simulink model "reichardt_array_EMD"  (R2018b)
settings: Solver=ode45  StartTime=0.0  StopTime=setStopTime  FixedStep=0.0005  RelTol=1e-3  EnableMultiTasking=on
model workspace (MAT data in the model file):
  bodyAmp = 0
  bodyPhase = 0
  freq = 628.318530718
  headAmp = 0
  headPhase = 0
  imageData = [0.00303351691359 0.00909998476947 0.0151647548087 0.0212266954775 0.0272846757084 0.0333375651143 0.0393842341832 0.0454235544723 0.0514543988027 0.0574756414532 0.0634861583552 0.0694848272865 ... (8204 elements, 1x8204)]
  outputTimeList = [1 1.0001 1.0002 1.0003 1.0004 1.0005 1.0006 1.0007 1.0008 1.0009 1.001 1.0011 ... (101 elements, 1x101)]
  setStopTime = 1.01
  stimAmp = 5
  temporalFilt = 0.046
  timeConstant = 0.046
libraries: visionsources x1
(part 2 of 2)

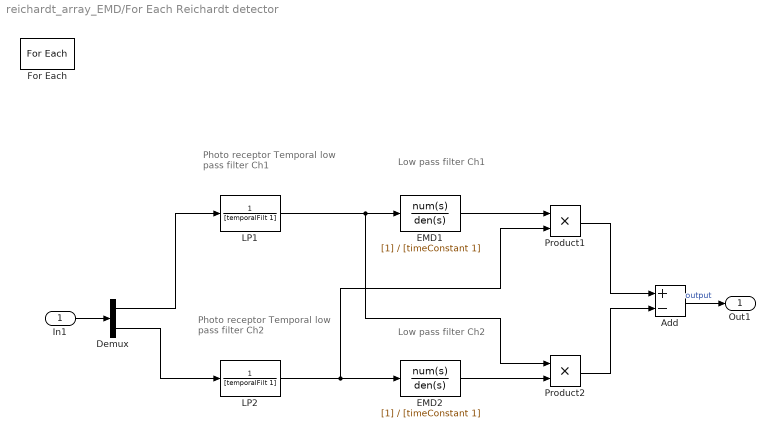
== system reichardt_array_EMD/For Each Reichardt detector ==
  note: Photo receptor
      | Temporal low pass filter
      | Ch2
  note: Photo receptor
      | Temporal low pass filter
      | Ch1
  note: Low pass filter
      | Ch1
  note: Low pass filter
      | Ch2
  In1 : Inport  Partition=on  PartitionDimension=1  PartitionWidth=1  PartitionOffset=0
  Add : Sum  Inputs=+-
  Demux : Demux  Outputs=2
  EMD1 : TransferFcn  Denominator=[timeConstant 1]
  EMD2 : TransferFcn  Denominator=[timeConstant 1]
  For Each : ForEach  DisableCoverage=on  IndexMode=One-based
  LP1 : TransferFcn  Numerator=1  Denominator=[temporalFilt 1]
  LP2 : TransferFcn  Numerator=1  Denominator=[temporalFilt 1]
  Product1 : Product  RndMeth=Zero
  Product2 : Product  RndMeth=Zero
  Out1 : Outport  ConcatenationDimension=1
  wires:
  EMD1/1 -> Product1/1
  Product1/1 -> Add/1
  Product2/1 -> Add/2
  EMD2/1 -> Product2/2
  Add/1 -> Out1/1  "output"
  Demux/1 -> LP1/1
  In1/1 -> Demux/1
  Demux/2 -> LP2/1
  LP2/1 -> EMD2/1, Product1/2
  LP1/1 -> EMD1/1, Product2/1

== matlab function reichardt_array_EMD/sampleImage ==
  data: imageData input; intensity output double size=360,2; seenAngle input
function intensity = fcn(imageData,seenAngle)
%#codegen

imageWidth = length(imageData);

% Subsample with resolution of compound eye
sampleCoord = 0:359;
sampleCoord = sampleCoord + seenAngle;
sampleCoord = mod(sampleCoord,360);
temp        = interp1(linspace(0,360,imageWidth),imageData,sampleCoord);

% Create output signals
intensity = [temp(:), circshift(temp(:),-1)];
